simulink model "initial_setup"  (R2012b)
settings: Solver=FixedStepDiscrete  StartTime=0.0  StopTime=inf  FixedStep=sample_time  RelTol=1e-3
InitFcn:
  | init_initial_setup;
values from neighbouring files (symbols this model uses):
  fcut_unwrap = 50    [init_initial_setup.m]
  fcut_velocity = 100    [init_initial_setup.m]
  sample_time = 1/update_freq    (= 0.001)    [init_initial_setup.m]
undefined symbols (not defined in the file or in its folder): A_angle_h, A_angle_k, A_angle_lat, angle_midpoint_h, angle_midpoint_k, angle_midpoint_lat, BOOM_MAX_ENCODER_TICKS, BOOM_PITCH_CAL_VALUE_RAD, BOOM_PITCH_CAL_VALUE_TICKS, BOOM_PITCH_ENCODER_RAD_PER_TICK, BOOM_ROLL_CAL_VALUE_RAD, BOOM_ROLL_CAL_VALUE_TICKS, BOOM_ROLL_ENCODER_RAD_PER_TICK, BOOM_YAW_ENCODER_RAD_PER_TICK, control_start_time, HIP_ABS_ENCODER_RAD_PER_TICK, HIP_INC_ENCODER_RAD_PER_TICK, HIP_INC_MAX_ENCODER_TICKS, k_leg_spring, kd_h_sine_walk, kd_k_sine_walk, kd_lat, kd_sea_position, kd_sea_torque, kd_velocity, kp_h_sine_walk, kp_k_sine_walk, kp_lat, kp_sea_position, kp_sea_torque, kp_velocity, LEFT_HIP_CALIB_POS, LEFT_HIP_CALIB_VAL, LEFT_MOTOR_HIP_DIRECTION, LEG1_LEG_A_CALIB_VAL, LEG1_LEG_A_RAD_PER_CNT, LEG1_LEG_B_CALIB_VAL, LEG1_LEG_B_RAD_PER_CNT, LEG1_MOTOR_A_DIRECTION, LEG1_MOTOR_B_DIRECTION, LEG1_TRAN_A_CALIB_VAL, LEG1_TRAN_A_RAD_PER_CNT, LEG1_TRAN_B_CALIB_VAL, LEG1_TRAN_B_RAD_PER_CNT, LEG2_LEG_A_CALIB_VAL, LEG2_LEG_A_RAD_PER_CNT, LEG2_LEG_B_CALIB_VAL, LEG2_LEG_B_RAD_PER_CNT, LEG2_MOTOR_A_DIRECTION, LEG2_MOTOR_B_DIRECTION, LEG2_TRAN_A_CALIB_VAL, LEG2_TRAN_A_RAD_PER_CNT, LEG2_TRAN_B_CALIB_VAL, LEG2_TRAN_B_RAD_PER_CNT, LEG_A_CALIB_LOC, LEG_B_CALIB_LOC, LEG_MTR_GEAR_RATIO, LEG_MTR_MAX_TORQUE, LEG_MTR_MAX_VELOCITY, MTR_HIP_MAX_CURRENT ... (+10)
libraries: xpcethercatlib x160, simulink x34, dspswit3 x1
(part 3 of 4)

== system initial_setup/Simple Sinusoidal Motion/SEA Controllers (Left Leg) ==
  phi_load_back : Inport
  phi_gear_back : Inport  Port=2
  phi_load_front : Inport  Port=3
  phi_gear_front : Inport  Port=4
  tau_des_back : Inport  Port=5
  tau_des_front : Inport  Port=6
  SEA Controller (Position) back : Subsystem
  SEA Controller (Position) front : Subsystem
  SEA Controller (Velocity) back : Subsystem  Commented=on
  SEA Controller (Velocity) front : Subsystem  Commented=on
  tau_cmd_back : Outport
  tau_cmd_front : Outport  Port=2
  wires:
  phi_load_front/1 -> SEA Controller (Position) front/1(phi_load [rad])
  tau_des_front/1 -> SEA Controller (Position) front/3(tau_des [Nm])
  SEA Controller (Position) back/1(tau_cmd [Nm]) -> tau_cmd_back/1
  phi_gear_back/1 -> SEA Controller (Position) back/2(phi_gear [rad])
  phi_gear_front/1 -> SEA Controller (Position) front/2(phi_gear [rad])
  phi_load_back/1 -> SEA Controller (Position) back/1(phi_load [rad])
  tau_des_back/1 -> SEA Controller (Position) back/3(tau_des [Nm])
  SEA Controller (Position) front/1(tau_cmd [Nm]) -> tau_cmd_front/1

== system initial_setup/Simple Sinusoidal Motion/SEA Controllers (Right Leg) ==
  phi_load_back : Inport
  phi_gear_back : Inport  Port=2
  phi_load_front : Inport  Port=3
  phi_gear_front : Inport  Port=4
  tau_des_back : Inport  Port=5
  tau_des_front : Inport  Port=6
  SEA Controller (Position) back : Subsystem
  SEA Controller (Position) front : Subsystem
  SEA Controller (Velocity) back : Subsystem  Commented=on
  SEA Controller (Velocity) front : Subsystem  Commented=on
  tau_cmd_back : Outport
  tau_cmd_front : Outport  Port=2
  wires:
  SEA Controller (Position) front/1(tau_cmd [Nm]) -> tau_cmd_front/1
  tau_des_back/1 -> SEA Controller (Position) back/3(tau_des [Nm])
  phi_load_back/1 -> SEA Controller (Position) back/1(phi_load [rad])
  phi_gear_front/1 -> SEA Controller (Position) front/2(phi_gear [rad])
  phi_gear_back/1 -> SEA Controller (Position) back/2(phi_gear [rad])
  SEA Controller (Position) back/1(tau_cmd [Nm]) -> tau_cmd_back/1
  tau_des_front/1 -> SEA Controller (Position) front/3(tau_des [Nm])
  phi_load_front/1 -> SEA Controller (Position) front/1(phi_load [rad])

== system initial_setup/DAQ/calibrate_and_convert_to_rad/calibrate_abs_encoder ==
  encoder_ticks : Inport
  cal_pt_ticks : Inport  Port=2
  cal_pt_rad : Inport  Port=3
  ticks_to_rad_const : Inport  Port=4
  Product : Product  RndMeth=Zero
  Sum : Sum  Inputs=|+-
  Sum1 : Sum  Inputs=|++
  angle [rad] : Outport
  wires:
  cal_pt_rad/1 -> Sum1/2  "calibration_point_radians"
  Sum1/1 -> angle [rad]/1  "calibrated_angle"
  cal_pt_ticks/1 -> Sum/2  "calibration_point_ticks"
  ticks_to_rad_const/1 -> Product/2  "ticks_to_rad_const"
  Product/1 -> Sum1/1  "rad_diff"
  encoder_ticks/1 -> Sum/1  "encoder_ticks"
  Sum/1 -> Product/1  "tick_diff"

== system initial_setup/DAQ/calibrate_and_convert_to_rad/calibration_pt_radians ==
  Constant{1,3,5,7} (4 alike) : Constant  Value=LEG_A_CALIB_LOC
  Constant10 : Constant  Value=LEFT_HIP_CALIB_POS
  Constant11 : Constant  Value=BOOM_ROLL_CAL_VALUE_RAD
  Constant12 : Constant  Value=BOOM_PITCH_CAL_VALUE_RAD
  Constant{2,4,6,8} (4 alike) : Constant  Value=LEG_B_CALIB_LOC
  Constant9 : Constant  Value=RIGHT_HIP_CALIB_POS
  Mux3 : Mux  Inputs=12
  calibration_pt [rad] : Outport
  wires:
  Constant7/1 -> Mux3/5
  Constant10/1 -> Mux3/9
  Constant1/1 -> Mux3/2
  Constant5/1 -> Mux3/6
  Constant2/1 -> Mux3/3
  Constant9/1 -> Mux3/10
  Constant12/1 -> Mux3/12
  Constant6/1 -> Mux3/7
  Constant11/1 -> Mux3/11
  Mux3/1 -> calibration_pt [rad]/1
  Constant3/1 -> Mux3/1
  Constant8/1 -> Mux3/8
  Constant4/1 -> Mux3/4

== system initial_setup/DAQ/calibrate_and_convert_to_rad/calibration_pt_ticks ==
  Constant1 : Constant  Value=LEG2_TRAN_A_CALIB_VAL
  Constant10 : Constant  Value=LEFT_HIP_CALIB_VAL
  Constant11 : Constant  Value=BOOM_ROLL_CAL_VALUE_TICKS
  Constant12 : Constant  Value=BOOM_PITCH_CAL_VALUE_TICKS
  Constant2 : Constant  Value=LEG2_LEG_B_CALIB_VAL
  Constant3 : Constant  Value=LEG2_LEG_A_CALIB_VAL
  Constant4 : Constant  Value=LEG2_TRAN_B_CALIB_VAL
  Constant5 : Constant  Value=LEG1_TRAN_A_CALIB_VAL
  Constant6 : Constant  Value=LEG1_LEG_B_CALIB_VAL
  Constant7 : Constant  Value=LEG1_LEG_A_CALIB_VAL
  Constant8 : Constant  Value=LEG1_TRAN_B_CALIB_VAL
  Constant9 : Constant  Value=RIGHT_HIP_CALIB_VAL
  Mux3 : Mux  Inputs=12
  calibration_pt [ticks] : Outport
  wires:
  Constant8/1 -> Mux3/4
  Constant4/1 -> Mux3/8
  Constant7/1 -> Mux3/1
  Mux3/1 -> calibration_pt [ticks]/1
  Constant11/1 -> Mux3/11
  Constant2/1 -> Mux3/7
  Constant12/1 -> Mux3/12
  Constant9/1 -> Mux3/10
  Constant6/1 -> Mux3/3
  Constant1/1 -> Mux3/6
  Constant5/1 -> Mux3/2
  Constant10/1 -> Mux3/9
  Constant3/1 -> Mux3/5

== system initial_setup/DAQ/calibrate_and_convert_to_rad/ticks_to_radians_constants ==
  Constant1 : Constant  Value=LEG2_TRAN_A_RAD_PER_CNT
  Constant10 : Constant  Value=-HIP_ABS_ENCODER_RAD_PER_TICK
  Constant11 : Constant  Value=BOOM_ROLL_ENCODER_RAD_PER_TICK
  Constant12 : Constant  Value=BOOM_PITCH_ENCODER_RAD_PER_TICK
  Constant2 : Constant  Value=LEG2_LEG_B_RAD_PER_CNT
  Constant3 : Constant  Value=LEG2_LEG_A_RAD_PER_CNT
  Constant4 : Constant  Value=LEG2_TRAN_B_RAD_PER_CNT
  Constant5 : Constant  Value=LEG1_TRAN_A_RAD_PER_CNT
  Constant6 : Constant  Value=LEG1_LEG_B_RAD_PER_CNT
  Constant7 : Constant  Value=LEG1_LEG_A_RAD_PER_CNT
  Constant8 : Constant  Value=LEG1_TRAN_B_RAD_PER_CNT
  Constant9 : Constant  Value=HIP_ABS_ENCODER_RAD_PER_TICK
  Mux3 : Mux  Inputs=12
  ticks_to_rad_constants : Outport
  wires:
  Constant8/1 -> Mux3/4
  Constant4/1 -> Mux3/8
  Constant7/1 -> Mux3/1
  Mux3/1 -> ticks_to_rad_constants/1
  Constant11/1 -> Mux3/11
  Constant2/1 -> Mux3/7
  Constant12/1 -> Mux3/12
  Constant10/1 -> Mux3/10
  Constant6/1 -> Mux3/3
  Constant1/1 -> Mux3/6
  Constant5/1 -> Mux3/2
  Constant9/1 -> Mux3/9
  Constant3/1 -> Mux3/5

== system initial_setup/DAQ/hold_initial_lateral_angles/Initial Lateral Hip Angles [rad] ==
  In : Inport
  Enable : EnablePort  StatesWhenEnabling=reset
  Out : Outport
  wires:
  In/1 -> Out/1

== system initial_setup/DAQ/unwrap_encoders/unwrap_boom_yaw_encoder ==
  note: predicted angle:
      | phi' = phi_(n-1) + dphi
      | = phi_(n-1) + phi_(n-1)-phi_(n-2)
  note: Transform Wrapped Angle into Continuous Angle
  note: Recommended if-then structure for assigning
      | constants. The criterion '~=0' is realized as cpu register
      | shift when compiling.  The resulting code is fast.
  wrapped [ticks] : Inport
  1/BOOM_MAX_ENCODER_TICKS : Gain  Gain=1/BOOM_MAX_ENCODER_TICKS
  Abs : Abs
  BOOM_MAX_ENCODER_TICKS : Gain  Gain=BOOM_MAX_ENCODER_TICKS
  Compare To Zero : simulink/Logic and Bit Operations/Compare To Zero  relop=>  OutDataTypeStr=uint8
  Discrete Single Pole Lowpass Filter : DiscreteTransferFcn  Numerator=[(1-exp(-2*pi*fcut_unwrap*sample_time)) 0]  Denominator=[1 -exp(-2*pi*fcut_unwrap*sample_time)]  SampleTime=sample_time
  Gain2 : Gain  Gain=2
  Product : Product  RndMeth=Zero
  Rounding Function : Rounding
  Sum : Sum  Inputs=|+-
  Sum1 : Sum  Inputs=|++
  Sum2 : Sum  Inputs=|++
  Sum3 : Sum  Inputs=-+|
  Switch : Switch  Criteria=u2 ~= 0
      settings: AttributesFormatString=%<Criteria>
  Unit Delay phi_(n-1) : UnitDelay  SampleTime=-1
      settings: AttributesFormatString=initial condition = %<X0>
  Unit Delay phi_(n-2) : UnitDelay  SampleTime=-1
      settings: AttributesFormatString=initial condition = %<X0>
  const : Constant  Value=0.5
  no : Constant  Value=-1
  yes : Constant
  continuous [ticks] : Outport
  wires:
  Sum3/1 -> Compare To Zero/1, Abs/1  "phi'-phi"
  Sum/1 -> Sum3/2
  Gain2/1 -> Sum/1
  Unit Delay phi_(n-1)/1 -> Gain2/1, Unit Delay phi_(n-2)/1
  BOOM_MAX_ENCODER_TICKS/1 -> Product/1
  Sum1/1 -> Discrete Single Pole Lowpass Filter/1, continuous [ticks]/1
  Sum2/1 -> Rounding Function/1
  const/1 -> Sum2/2
  1/BOOM_MAX_ENCODER_TICKS/1 -> Sum2/1
  Abs/1 -> 1/BOOM_MAX_ENCODER_TICKS/1
  Product/1 -> Sum1/2
  wrapped [ticks]/1 -> Sum3/1, Sum1/1
  Rounding Function/1 -> BOOM_MAX_ENCODER_TICKS/1
  Switch/1 -> Product/2
  no/1 -> Switch/3
  yes/1 -> Switch/1
  Unit Delay phi_(n-2)/1 -> Sum/2
  Compare To Zero/1 -> Switch/2
  Discrete Single Pole Lowpass Filter/1 -> Unit Delay phi_(n-1)/1

== system initial_setup/DAQ/unwrap_encoders/unwrap_lateral_incremental_encoders Left ==
  note: predicted angle:
      | phi' = phi_(n-1) + dphi
      | = phi_(n-1) + phi_(n-1)-phi_(n-2)
  note: Transform Wrapped Angle into Continuous Angle
  note: Recommended if-then structure for assigning
      | constants. The criterion '~=0' is realized as cpu register
      | shift when compiling.  The resulting code is fast.
  wrapped [ticks] : Inport
  1/HIP_INC_MAX_ENCODER_TICKS : Gain  Gain=1/HIP_INC_MAX_ENCODER_TICKS
  Abs : Abs
  Compare To Zero : simulink/Logic and Bit Operations/Compare To Zero  relop=>  OutDataTypeStr=uint8
  Discrete Single Pole Lowpass Filter : DiscreteTransferFcn  Numerator=[(1-exp(-2*pi*fcut_unwrap*sample_time)) 0]  Denominator=[1 -exp(-2*pi*fcut_unwrap*sample_time)]  SampleTime=sample_time
  Gain2 : Gain  Gain=2
  HIP_INC_MAX_ENCODER_TICKS : Gain  Gain=HIP_INC_MAX_ENCODER_TICKS
  Product : Product  RndMeth=Zero
  Rounding Function : Rounding
  Sum : Sum  Inputs=|+-
  Sum1 : Sum  Inputs=|++
  Sum2 : Sum  Inputs=|++
  Sum3 : Sum  Inputs=-+|
  Switch : Switch  Criteria=u2 ~= 0
      settings: AttributesFormatString=%<Criteria>
  Unit Delay phi_(n-1) : UnitDelay  SampleTime=-1
      settings: AttributesFormatString=initial condition = %<X0>
  Unit Delay phi_(n-2) : UnitDelay  SampleTime=-1
      settings: AttributesFormatString=initial condition = %<X0>
  const : Constant  Value=0.5
  no : Constant  Value=-1
  yes : Constant
  continuous [ticks] : Outport
  wires:
  Sum3/1 -> Compare To Zero/1, Abs/1  "phi'-phi"
  Sum/1 -> Sum3/2
  Gain2/1 -> Sum/1
  Unit Delay phi_(n-1)/1 -> Gain2/1, Unit Delay phi_(n-2)/1
  HIP_INC_MAX_ENCODER_TICKS/1 -> Product/1
  Sum1/1 -> continuous [ticks]/1, Discrete Single Pole Lowpass Filter/1
  Sum2/1 -> Rounding Function/1
  const/1 -> Sum2/2
  1/HIP_INC_MAX_ENCODER_TICKS/1 -> Sum2/1
  Abs/1 -> 1/HIP_INC_MAX_ENCODER_TICKS/1
  Product/1 -> Sum1/2
  wrapped [ticks]/1 -> Sum3/1, Sum1/1
  Rounding Function/1 -> HIP_INC_MAX_ENCODER_TICKS/1
  Switch/1 -> Product/2
  no/1 -> Switch/3
  yes/1 -> Switch/1
  Unit Delay phi_(n-2)/1 -> Sum/2
  Compare To Zero/1 -> Switch/2
  Discrete Single Pole Lowpass Filter/1 -> Unit Delay phi_(n-1)/1

== system initial_setup/DAQ/unwrap_encoders/unwrap_lateral_incremental_encoders Right ==
  note: Recommended if-then structure for assigning
      | constants. The criterion '~=0' is realized as cpu register
      | shift when compiling.  The resulting code is fast.
  note: Transform Wrapped Angle into Continuous Angle
  note: predicted angle:
      | phi' = phi_(n-1) + dphi
      | = phi_(n-1) + phi_(n-1)-phi_(n-2)
  wrapped [ticks] : Inport
  1/HIP_INC_MAX_ENCODER_TICKS : Gain  Gain=1/HIP_INC_MAX_ENCODER_TICKS
  Abs : Abs
  Compare To Zero : simulink/Logic and Bit Operations/Compare To Zero  relop=>  OutDataTypeStr=uint8
  Discrete Single Pole Lowpass Filter : DiscreteTransferFcn  Numerator=[(1-exp(-2*pi*fcut_unwrap*sample_time)) 0]  Denominator=[1 -exp(-2*pi*fcut_unwrap*sample_time)]  SampleTime=sample_time
  Gain2 : Gain  Gain=2
  HIP_INC_MAX_ENCODER_TICKS : Gain  Gain=HIP_INC_MAX_ENCODER_TICKS
  Product : Product  RndMeth=Zero
  Rounding Function : Rounding
  Sum : Sum  Inputs=|+-
  Sum1 : Sum  Inputs=|++
  Sum2 : Sum  Inputs=|++
  Sum3 : Sum  Inputs=-+|
  Switch : Switch  Criteria=u2 ~= 0
      settings: AttributesFormatString=%<Criteria>
  Unit Delay phi_(n-1) : UnitDelay  SampleTime=-1
      settings: AttributesFormatString=initial condition = %<X0>
  Unit Delay phi_(n-2) : UnitDelay  SampleTime=-1
      settings: AttributesFormatString=initial condition = %<X0>
  const : Constant  Value=0.5
  no : Constant  Value=-1
  yes : Constant
  continuous [ticks] : Outport
  wires:
  Discrete Single Pole Lowpass Filter/1 -> Unit Delay phi_(n-1)/1
  Compare To Zero/1 -> Switch/2
  Unit Delay phi_(n-2)/1 -> Sum/2
  yes/1 -> Switch/1
  no/1 -> Switch/3
  Switch/1 -> Product/2
  Rounding Function/1 -> HIP_INC_MAX_ENCODER_TICKS/1
  wrapped [ticks]/1 -> Sum1/1, Sum3/1
  Product/1 -> Sum1/2
  Abs/1 -> 1/HIP_INC_MAX_ENCODER_TICKS/1
  1/HIP_INC_MAX_ENCODER_TICKS/1 -> Sum2/1
  const/1 -> Sum2/2
  Sum2/1 -> Rounding Function/1
  Sum1/1 -> Discrete Single Pole Lowpass Filter/1, continuous [ticks]/1
  HIP_INC_MAX_ENCODER_TICKS/1 -> Product/1
  Unit Delay phi_(n-1)/1 -> Unit Delay phi_(n-2)/1, Gain2/1
  Gain2/1 -> Sum/1
  Sum/1 -> Sum3/2
  Sum3/1 -> Abs/1, Compare To Zero/1  "phi'-phi"

== system initial_setup/Simple Sinusoidal Motion/Left Lateral Sine Wave/Diminish ==
  desQ : Inport
  Clock : Clock
  Divide : Product  Inputs=*/
  Position Saturation : Saturate  UpperLimit=0  LowerLimit=-5*pi/180
  Ramp : simulink/Sources/Ramp  slope=pi/10  start=t_lat  X0=1
  Ramp1 : simulink/Sources/Ramp  slope=-0.5*pi/180  start=t_lat  X0=0
  Sum : Sum  Inputs=++|
  Switch : Switch  Threshold=t_lat
  desQ' : Outport
  wires:
  Clock/1 -> Switch/2
  Ramp/1 -> Divide/2
  Switch/1 -> desQ'/1
  desQ/1 -> Switch/3, Divide/1
  Ramp1/1 -> Position Saturation/1
  Divide/1 -> Sum/2
  Position Saturation/1 -> Sum/1
  Sum/1 -> Switch/1

== system initial_setup/Simple Sinusoidal Motion/Left Lateral Sine Wave/Hip Roll PD ==
  Desired Position / Velocity : Inport
  Position / Velocity : Inport  Port=2
  Demux : Demux  Outputs=2
  Demux1 : Demux  Outputs=2
  Gain4 : Gain  Gain=kp_lat
  Gain5 : Gain  Gain=kd_lat
  Sum4 : Sum  Inputs=|+-
  Sum5 : Sum  Inputs=|+-
  Sum6 : Sum  Inputs=|++
  tauLat : Outport
  wires:
  Sum6/1 -> tauLat/1
  Demux/1 -> Sum4/2  "position"
  Position / Velocity/1 -> Demux/1
  Sum4/1 -> Gain4/1
  Sum5/1 -> Gain5/1
  Gain4/1 -> Sum6/1
  Demux/2 -> Sum5/2  "velocity"
  Gain5/1 -> Sum6/2
  Demux1/2 -> Sum5/1
  Desired Position / Velocity/1 -> Demux1/1
  Demux1/1 -> Sum4/1

== system initial_setup/Simple Sinusoidal Motion/Left Leg Sagittal Sine Wave/Hip PD Torque Control ==
  Desired Angle : Inport
  Desired Velocity : Inport  Port=2
  Hip Position / Velocity : Inport  Port=3
  Demux : Demux  Outputs=2
  Gain4 : Gain  Gain=kp_h_sine_walk
  Gain5 : Gain  Gain=kd_h_sine_walk
  Sum4 : Sum  Inputs=|+-
  Sum5 : Sum  Inputs=|+-
  Sum6 : Sum  Inputs=|++
  Tau Hip : Outport
  wires:
  Gain5/1 -> Sum6/2
  Demux/2 -> Sum5/2  "theta_h_dot_measured"
  Gain4/1 -> Sum6/1
  Sum5/1 -> Gain5/1
  Sum4/1 -> Gain4/1
  Desired Velocity/1 -> Sum5/1
  Hip Position / Velocity/1 -> Demux/1
  Demux/1 -> Sum4/2  "theta_h_measured"
  Desired Angle/1 -> Sum4/1
  Sum6/1 -> Tau Hip/1

== system initial_setup/Simple Sinusoidal Motion/Left Leg Sagittal Sine Wave/Knee PD Torque Control ==
  Desired Angle : Inport
  Desired Velocity : Inport  Port=2
  Knee Position / Velocity : Inport  Port=3
  Demux1 : Demux  Outputs=2
  Gain6 : Gain  Gain=kp_k_sine_walk
  Gain7 : Gain  Gain=kd_k_sine_walk
  Sum7 : Sum  Inputs=|+-
  Sum8 : Sum  Inputs=|+-
  Sum9 : Sum  Inputs=|++
  Tau Knee : Outport
  wires:
  Gain6/1 -> Sum9/1
  Gain7/1 -> Sum9/2
  Knee Position / Velocity/1 -> Demux1/1
  Demux1/2 -> Sum8/2  "theta_k_dot_measured"
  Desired Angle/1 -> Sum7/1
  Sum8/1 -> Gain7/1
  Desired Velocity/1 -> Sum8/1
  Sum9/1 -> Tau Knee/1
  Demux1/1 -> Sum7/2  "theta_k_measured"
  Sum7/1 -> Gain6/1

== system initial_setup/Simple Sinusoidal Motion/Right Lateral Sine Wave/Diminish ==
  desQ : Inport
  Clock : Clock
  Divide : Product  Inputs=*/
  Position Saturation : Saturate  UpperLimit=0  LowerLimit=-5*pi/180
  Ramp : simulink/Sources/Ramp  slope=-0.5*pi/180  start=t_lat  X0=0
  Ramp1 : simulink/Sources/Ramp  slope=pi/10  start=t_lat  X0=1
  Sum : Sum  Inputs=++|
  Switch : Switch  Threshold=t_lat
  desQ' : Outport
  wires:
  Clock/1 -> Switch/2
  Ramp1/1 -> Divide/2
  Switch/1 -> desQ'/1
  desQ/1 -> Switch/3, Divide/1
  Ramp/1 -> Position Saturation/1
  Divide/1 -> Sum/2
  Sum/1 -> Switch/1
  Position Saturation/1 -> Sum/1

== system initial_setup/Simple Sinusoidal Motion/Right Lateral Sine Wave/Hip Roll PD ==
  Desired Position / Velocity : Inport
  Position / Velocity : Inport  Port=2
  Demux : Demux  Outputs=2
  Demux1 : Demux  Outputs=2
  Gain4 : Gain  Gain=kp_lat
  Gain5 : Gain  Gain=kd_lat
  Sum4 : Sum  Inputs=|+-
  Sum5 : Sum  Inputs=|+-
  Sum6 : Sum  Inputs=|++
  tauLat : Outport
  wires:
  Gain5/1 -> Sum6/2
  Demux/2 -> Sum5/2  "velocity"
  Gain4/1 -> Sum6/1
  Sum5/1 -> Gain5/1
  Sum4/1 -> Gain4/1
  Demux1/2 -> Sum5/1
  Position / Velocity/1 -> Demux/1
  Demux/1 -> Sum4/2  "position"
  Desired Position / Velocity/1 -> Demux1/1
  Sum6/1 -> tauLat/1
  Demux1/1 -> Sum4/1

== system initial_setup/Simple Sinusoidal Motion/Right Leg Sagittal Sine Wave/Hip PD Torque Control ==
  Desired Angle : Inport
  Desired Velocity : Inport  Port=2
  Hip Position / Velocity : Inport  Port=3
  Demux : Demux  Outputs=2
  Gain4 : Gain  Gain=kp_h_sine_walk
  Gain5 : Gain  Gain=kd_h_sine_walk
  Sum4 : Sum  Inputs=|+-
  Sum5 : Sum  Inputs=|+-
  Sum6 : Sum  Inputs=|++
  Tau Hip : Outport
  wires:
  Sum6/1 -> Tau Hip/1
  Desired Angle/1 -> Sum4/1
  Demux/1 -> Sum4/2  "theta_h_measured"
  Hip Position / Velocity/1 -> Demux/1
  Desired Velocity/1 -> Sum5/1
  Sum4/1 -> Gain4/1
  Sum5/1 -> Gain5/1
  Gain4/1 -> Sum6/1
  Demux/2 -> Sum5/2  "theta_h_dot_measured"
  Gain5/1 -> Sum6/2

== system initial_setup/Simple Sinusoidal Motion/Right Leg Sagittal Sine Wave/Knee PD Torque Control ==
  Desired Angle : Inport
  Desired Velocity : Inport  Port=2
  Knee Position / Velocity : Inport  Port=3
  Demux1 : Demux  Outputs=2
  Gain6 : Gain  Gain=kp_k_sine_walk
  Gain7 : Gain  Gain=kd_k_sine_walk
  Sum7 : Sum  Inputs=|+-
  Sum8 : Sum  Inputs=|+-
  Sum9 : Sum  Inputs=|++
  Tau Knee : Outport
  wires:
  Sum7/1 -> Gain6/1
  Demux1/1 -> Sum7/2  "theta_k_measured"
  Sum9/1 -> Tau Knee/1
  Desired Velocity/1 -> Sum8/1
  Sum8/1 -> Gain7/1
  Desired Angle/1 -> Sum7/1
  Demux1/2 -> Sum8/2  "theta_k_dot_measured"
  Knee Position / Velocity/1 -> Demux1/1
  Gain7/1 -> Sum9/2
  Gain6/1 -> Sum9/1

== system initial_setup/Simple Sinusoidal Motion/SEA Controllers (Left Leg)/SEA Controller (Position) back ==
  phi_load [rad] : Inport
  phi_gear [rad] : Inport  Port=2
  tau_des [Nm] : Inport  Port=3
  Gain2 : Gain  Gain=1/k_leg_spring
  Position PD : Subsystem
  Spring Stiffness : Gain  Gain=k_leg_spring
  Sum1 : Sum  Inputs=+-
  Sum2 : Sum  Inputs=|+-
  Sum3 : Sum  Inputs=+|+
  Sum4 : Sum  Inputs=|+-
  Sum5 : Sum  Inputs=++|
  "Torque Limiter (outside) " : Saturate  UpperLimit=LEG_MTR_MAX_TORQUE  LowerLimit=-LEG_MTR_MAX_TORQUE
  Torque PD : Subsystem
  tau_cmd [Nm] : Outport
  wires:
  phi_gear [rad]/1 -> Sum1/1, Sum4/2
  Sum4/1 -> Position PD/1(position_Err)
  Position PD/1(out) -> tau_cmd [Nm]/1
  "Torque Limiter (outside) "/1 -> Sum2/1, Gain2/1
  Gain2/1 -> Sum3/1
  Spring Stiffness/1 -> Sum2/2  "tau_L"
  tau_des [Nm]/1 -> "Torque Limiter (outside) "/1
  Sum2/1 -> Torque PD/1(tau_Err)  "tau_Err"
  Sum1/1 -> Spring Stiffness/1
  phi_load [rad]/1 -> Sum3/2, Sum1/2
  Sum3/1 -> Sum5/1
  Sum5/1 -> Sum4/1
  Torque PD/1(out) -> Sum5/2

== system initial_setup/Simple Sinusoidal Motion/SEA Controllers (Left Leg)/SEA Controller (Position) front ==
  phi_load [rad] : Inport
  phi_gear [rad] : Inport  Port=2
  tau_des [Nm] : Inport  Port=3
  Gain2 : Gain  Gain=1/k_leg_spring
  Position PD : Subsystem
  Spring Stiffness : Gain  Gain=k_leg_spring
  Sum1 : Sum  Inputs=+-
  Sum2 : Sum  Inputs=|+-
  Sum3 : Sum  Inputs=+|+
  Sum4 : Sum  Inputs=|+-
  Sum5 : Sum  Inputs=++|
  "Torque Limiter (outside) " : Saturate  UpperLimit=LEG_MTR_MAX_TORQUE  LowerLimit=-LEG_MTR_MAX_TORQUE
  Torque PD : Subsystem
  tau_cmd [Nm] : Outport
  wires:
  Torque PD/1(out) -> Sum5/2
  Sum5/1 -> Sum4/1
  Sum3/1 -> Sum5/1
  phi_load [rad]/1 -> Sum1/2, Sum3/2
  Sum1/1 -> Spring Stiffness/1
  Sum2/1 -> Torque PD/1(tau_Err)  "tau_Err"
  tau_des [Nm]/1 -> "Torque Limiter (outside) "/1
  Spring Stiffness/1 -> Sum2/2  "tau_L"
  Gain2/1 -> Sum3/1
  "Torque Limiter (outside) "/1 -> Gain2/1, Sum2/1
  Position PD/1(out) -> tau_cmd [Nm]/1
  Sum4/1 -> Position PD/1(position_Err)
  phi_gear [rad]/1 -> Sum4/2, Sum1/1

== system initial_setup/Simple Sinusoidal Motion/SEA Controllers (Left Leg)/SEA Controller (Velocity) back ==
  note: Feedback Error Compensation
  note: SEA
      | Electromechanical
      | Process
      | Dynamics
  note: Inverse Dynamics Compensation
  note: Anticipatory Feedforward Compensation
  phi_load [rad] : Inport
  phi_gear [rad] : Inport  Port=2
  tau_des [Nm] : Inport  Port=3
  1st Lead Compensator : Subsystem
  Gain2 : Gain  Gain=1/k_leg_spring
  Gear Ratio2 : Gain  Gain=LEG_MTR_GEAR_RATIO
  Lead Compensator : Subsystem
  PD : Subsystem
  PID : Subsystem
  Spring Stiffness : Gain  Gain=k_leg_spring
  Sum1 : Sum  Inputs=+-
  Sum2 : Sum  Inputs=|+-
  Sum3 : Sum  Inputs=+|+
  Sum4 : Sum  Inputs=|+-
  Sum5 : Sum  Inputs=++|
  "Torque Limiter (outside) " : Saturate  UpperLimit=LEG_MTR_MAX_TORQUE  LowerLimit=-LEG_MTR_MAX_TORQUE
  Velocity Limiter : Saturate  UpperLimit=LEG_MTR_MAX_VELOCITY  LowerLimit=-LEG_MTR_MAX_VELOCITY
  filtered_derivative : Subsystem
  tau_cmd [Nm] : Outport
  wires:
  PD/1(tau_mtr [Nm]) -> tau_cmd [Nm]/1
  Sum3/1 -> Sum5/1
  Gear Ratio2/1 -> Sum4/2
  filtered_derivative/1(dx/dt) -> Gear Ratio2/1
  Sum4/1 -> PD/1(velocity_err [rad/s])
  Velocity Limiter/1 -> Sum4/1
  Lead Compensator/1(dx/dt) -> Sum3/2
  "Torque Limiter (outside) "/1 -> Gain2/1, Sum2/1
  Sum5/1 -> Velocity Limiter/1  "dphi_gearhead_des  [m/s]"
  phi_gear [rad]/1 -> Sum1/1, filtered_derivative/1(x)
  1st Lead Compensator/1(dx/dt) -> Sum3/1
  PID/1("dphi_gearhead_des [rad/s] ") -> Sum5/2
  Spring Stiffness/1 -> Sum2/2  "tau_L"
  tau_des [Nm]/1 -> "Torque Limiter (outside) "/1
  Sum2/1 -> PID/1(tau_Err)  "tau_Err"
  Sum1/1 -> Spring Stiffness/1
  phi_load [rad]/1 -> Sum1/2, Lead Compensator/1(x)
  Gain2/1 -> 1st Lead Compensator/1(x)

== system initial_setup/Simple Sinusoidal Motion/SEA Controllers (Left Leg)/SEA Controller (Velocity) front ==
  note: Anticipatory Feedforward Compensation
  note: Inverse Dynamics Compensation
  note: SEA
      | Electromechanical
      | Process
      | Dynamics
  note: Feedback Error Compensation
  phi_load [rad] : Inport
  phi_gear [rad] : Inport  Port=2
  tau_des [Nm] : Inport  Port=3
  1st Lead Compensator : Subsystem
  Gain2 : Gain  Gain=1/k_leg_spring
  Gear Ratio2 : Gain  Gain=LEG_MTR_GEAR_RATIO
  Lead Compensator : Subsystem
  PD : Subsystem
  PID : Subsystem
  Spring Stiffness : Gain  Gain=k_leg_spring
  Sum1 : Sum  Inputs=+-
  Sum2 : Sum  Inputs=|+-
  Sum3 : Sum  Inputs=+|+
  Sum4 : Sum  Inputs=|+-
  Sum5 : Sum  Inputs=++|
  "Torque Limiter (outside) " : Saturate  UpperLimit=LEG_MTR_MAX_TORQUE  LowerLimit=-LEG_MTR_MAX_TORQUE
  Velocity Limiter : Saturate  UpperLimit=LEG_MTR_MAX_VELOCITY  LowerLimit=-LEG_MTR_MAX_VELOCITY
  filtered_derivative : Subsystem
  tau_cmd [Nm] : Outport
  wires:
  Gain2/1 -> 1st Lead Compensator/1(x)
  phi_load [rad]/1 -> Lead Compensator/1(x), Sum1/2
  Sum1/1 -> Spring Stiffness/1
  Sum2/1 -> PID/1(tau_Err)  "tau_Err"
  tau_des [Nm]/1 -> "Torque Limiter (outside) "/1
  Spring Stiffness/1 -> Sum2/2  "tau_L"
  PID/1("dphi_gearhead_des [rad/s] ") -> Sum5/2
  1st Lead Compensator/1(dx/dt) -> Sum3/1
  phi_gear [rad]/1 -> filtered_derivative/1(x), Sum1/1
  Sum5/1 -> Velocity Limiter/1  "dphi_gearhead_des  [m/s]"
  "Torque Limiter (outside) "/1 -> Sum2/1, Gain2/1
  Lead Compensator/1(dx/dt) -> Sum3/2
  Velocity Limiter/1 -> Sum4/1
  Sum4/1 -> PD/1(velocity_err [rad/s])
  filtered_derivative/1(dx/dt) -> Gear Ratio2/1
  Gear Ratio2/1 -> Sum4/2
  Sum3/1 -> Sum5/1
  PD/1(tau_mtr [Nm]) -> tau_cmd [Nm]/1

== system initial_setup/Simple Sinusoidal Motion/SEA Controllers (Right Leg)/SEA Controller (Position) back ==
  phi_load [rad] : Inport
  phi_gear [rad] : Inport  Port=2
  tau_des [Nm] : Inport  Port=3
  Gain2 : Gain  Gain=1/k_leg_spring
  Position PD : Subsystem
  Spring Stiffness : Gain  Gain=k_leg_spring
  Sum1 : Sum  Inputs=+-
  Sum2 : Sum  Inputs=|+-
  Sum3 : Sum  Inputs=+|+
  Sum4 : Sum  Inputs=|+-
  Sum5 : Sum  Inputs=++|
  "Torque Limiter (outside) " : Saturate  UpperLimit=LEG_MTR_MAX_TORQUE  LowerLimit=-LEG_MTR_MAX_TORQUE
  Torque PD : Subsystem
  tau_cmd [Nm] : Outport
  wires:
  Torque PD/1(out) -> Sum5/2
  Sum5/1 -> Sum4/1
  Sum3/1 -> Sum5/1
  phi_load [rad]/1 -> Sum1/2, Sum3/2
  Sum1/1 -> Spring Stiffness/1
  Sum2/1 -> Torque PD/1(tau_Err)  "tau_Err"
  tau_des [Nm]/1 -> "Torque Limiter (outside) "/1
  Spring Stiffness/1 -> Sum2/2  "tau_L"
  Gain2/1 -> Sum3/1
  "Torque Limiter (outside) "/1 -> Gain2/1, Sum2/1
  Position PD/1(out) -> tau_cmd [Nm]/1
  Sum4/1 -> Position PD/1(position_Err)
  phi_gear [rad]/1 -> Sum4/2, Sum1/1

== system initial_setup/Simple Sinusoidal Motion/SEA Controllers (Right Leg)/SEA Controller (Position) front ==
  phi_load [rad] : Inport
  phi_gear [rad] : Inport  Port=2
  tau_des [Nm] : Inport  Port=3
  Gain2 : Gain  Gain=1/k_leg_spring
  Position PD : Subsystem
  Spring Stiffness : Gain  Gain=k_leg_spring
  Sum1 : Sum  Inputs=+-
  Sum2 : Sum  Inputs=|+-
  Sum3 : Sum  Inputs=+|+
  Sum4 : Sum  Inputs=|+-
  Sum5 : Sum  Inputs=++|
  "Torque Limiter (outside) " : Saturate  UpperLimit=LEG_MTR_MAX_TORQUE  LowerLimit=-LEG_MTR_MAX_TORQUE
  Torque PD : Subsystem
  tau_cmd [Nm] : Outport
  wires:
  phi_gear [rad]/1 -> Sum1/1, Sum4/2
  Sum4/1 -> Position PD/1(position_Err)
  Position PD/1(out) -> tau_cmd [Nm]/1
  "Torque Limiter (outside) "/1 -> Sum2/1, Gain2/1
  Gain2/1 -> Sum3/1
  Spring Stiffness/1 -> Sum2/2  "tau_L"
  tau_des [Nm]/1 -> "Torque Limiter (outside) "/1
  Sum2/1 -> Torque PD/1(tau_Err)  "tau_Err"
  Sum1/1 -> Spring Stiffness/1
  phi_load [rad]/1 -> Sum3/2, Sum1/2
  Sum3/1 -> Sum5/1
  Sum5/1 -> Sum4/1
  Torque PD/1(out) -> Sum5/2

== system initial_setup/Simple Sinusoidal Motion/SEA Controllers (Right Leg)/SEA Controller (Velocity) back ==
  note: Anticipatory Feedforward Compensation
  note: Inverse Dynamics Compensation
  note: SEA
      | Electromechanical
      | Process
      | Dynamics
  note: Feedback Error Compensation
  phi_load [rad] : Inport
  phi_gear [rad] : Inport  Port=2
  tau_des [Nm] : Inport  Port=3
  1st Lead Compensator : Subsystem
  Gain2 : Gain  Gain=1/k_leg_spring
  Gear Ratio2 : Gain  Gain=LEG_MTR_GEAR_RATIO
  Lead Compensator : Subsystem
  PD : Subsystem
  PID : Subsystem
  Spring Stiffness : Gain  Gain=k_leg_spring
  Sum1 : Sum  Inputs=+-
  Sum2 : Sum  Inputs=|+-
  Sum3 : Sum  Inputs=+|+
  Sum4 : Sum  Inputs=|+-
  Sum5 : Sum  Inputs=++|
  "Torque Limiter (outside) " : Saturate  UpperLimit=LEG_MTR_MAX_TORQUE  LowerLimit=-LEG_MTR_MAX_TORQUE
  Velocity Limiter : Saturate  UpperLimit=LEG_MTR_MAX_VELOCITY  LowerLimit=-LEG_MTR_MAX_VELOCITY
  filtered_derivative : Subsystem
  tau_cmd [Nm] : Outport
  wires:
  Gain2/1 -> 1st Lead Compensator/1(x)
  phi_load [rad]/1 -> Lead Compensator/1(x), Sum1/2
  Sum1/1 -> Spring Stiffness/1
  Sum2/1 -> PID/1(tau_Err)  "tau_Err"
  tau_des [Nm]/1 -> "Torque Limiter (outside) "/1
  Spring Stiffness/1 -> Sum2/2  "tau_L"
  PID/1("dphi_gearhead_des [rad/s] ") -> Sum5/2
  1st Lead Compensator/1(dx/dt) -> Sum3/1
  phi_gear [rad]/1 -> filtered_derivative/1(x), Sum1/1
  Sum5/1 -> Velocity Limiter/1  "dphi_gearhead_des  [m/s]"
  "Torque Limiter (outside) "/1 -> Sum2/1, Gain2/1
  Lead Compensator/1(dx/dt) -> Sum3/2
  Velocity Limiter/1 -> Sum4/1
  Sum4/1 -> PD/1(velocity_err [rad/s])
  filtered_derivative/1(dx/dt) -> Gear Ratio2/1
  Gear Ratio2/1 -> Sum4/2
  Sum3/1 -> Sum5/1
  PD/1(tau_mtr [Nm]) -> tau_cmd [Nm]/1

== system initial_setup/Simple Sinusoidal Motion/SEA Controllers (Right Leg)/SEA Controller (Velocity) front ==
  note: Feedback Error Compensation
  note: SEA
      | Electromechanical
      | Process
      | Dynamics
  note: Inverse Dynamics Compensation
  note: Anticipatory Feedforward Compensation
  phi_load [rad] : Inport
  phi_gear [rad] : Inport  Port=2
  tau_des [Nm] : Inport  Port=3
  1st Lead Compensator : Subsystem
  Gain2 : Gain  Gain=1/k_leg_spring
  Gear Ratio2 : Gain  Gain=LEG_MTR_GEAR_RATIO
  Lead Compensator : Subsystem
  PD : Subsystem
  PID : Subsystem
  Spring Stiffness : Gain  Gain=k_leg_spring
  Sum1 : Sum  Inputs=+-
  Sum2 : Sum  Inputs=|+-
  Sum3 : Sum  Inputs=+|+
  Sum4 : Sum  Inputs=|+-
  Sum5 : Sum  Inputs=++|
  "Torque Limiter (outside) " : Saturate  UpperLimit=LEG_MTR_MAX_TORQUE  LowerLimit=-LEG_MTR_MAX_TORQUE
  Velocity Limiter : Saturate  UpperLimit=LEG_MTR_MAX_VELOCITY  LowerLimit=-LEG_MTR_MAX_VELOCITY
  filtered_derivative : Subsystem
  tau_cmd [Nm] : Outport
  wires:
  PD/1(tau_mtr [Nm]) -> tau_cmd [Nm]/1
  Sum3/1 -> Sum5/1
  Gear Ratio2/1 -> Sum4/2
  filtered_derivative/1(dx/dt) -> Gear Ratio2/1
  Sum4/1 -> PD/1(velocity_err [rad/s])
  Velocity Limiter/1 -> Sum4/1
  Lead Compensator/1(dx/dt) -> Sum3/2
  "Torque Limiter (outside) "/1 -> Gain2/1, Sum2/1
  Sum5/1 -> Velocity Limiter/1  "dphi_gearhead_des  [m/s]"
  phi_gear [rad]/1 -> Sum1/1, filtered_derivative/1(x)
  1st Lead Compensator/1(dx/dt) -> Sum3/1
  PID/1("dphi_gearhead_des [rad/s] ") -> Sum5/2
  Spring Stiffness/1 -> Sum2/2  "tau_L"
  tau_des [Nm]/1 -> "Torque Limiter (outside) "/1
  Sum2/1 -> PID/1(tau_Err)  "tau_Err"
  Sum1/1 -> Spring Stiffness/1
  phi_load [rad]/1 -> Sum1/2, Lead Compensator/1(x)
  Gain2/1 -> 1st Lead Compensator/1(x)

== system initial_setup/Simple Sinusoidal Motion/SEA Controllers (Left Leg)/SEA Controller (Position) back/Position PD ==
  position_Err : Inport
  Proportional Gain : Gain  Gain=kp_sea_position
  Proportional Gain1 : Gain  Gain=kd_sea_position
  Sum : Sum
  filtered_derivative : Subsystem
  out : Outport
  wires:
  filtered_derivative/1(dx/dt) -> Proportional Gain1/1
  Proportional Gain1/1 -> Sum/1
  Proportional Gain/1 -> Sum/2
  position_Err/1 -> Proportional Gain/1, filtered_derivative/1(x)
  Sum/1 -> out/1

== system initial_setup/Simple Sinusoidal Motion/SEA Controllers (Left Leg)/SEA Controller (Position) back/Torque PD ==
  tau_Err : Inport
  Proportional Gain : Gain  Gain=kp_sea_torque
  out : Outport
  wires:
  Proportional Gain/1 -> out/1
  tau_Err/1 -> Proportional Gain/1

== system initial_setup/Simple Sinusoidal Motion/SEA Controllers (Left Leg)/SEA Controller (Position) front/Position PD ==
  position_Err : Inport
  Proportional Gain : Gain  Gain=kp_sea_position
  Proportional Gain1 : Gain  Gain=kd_sea_position
  Sum : Sum
  filtered_derivative : Subsystem
  out : Outport
  wires:
  filtered_derivative/1(dx/dt) -> Proportional Gain1/1
  Sum/1 -> out/1
  position_Err/1 -> Proportional Gain/1, filtered_derivative/1(x)
  Proportional Gain/1 -> Sum/2
  Proportional Gain1/1 -> Sum/1

== system initial_setup/Simple Sinusoidal Motion/SEA Controllers (Left Leg)/SEA Controller (Position) front/Torque PD ==
  tau_Err : Inport
  Proportional Gain : Gain  Gain=kp_sea_torque
  out : Outport
  wires:
  tau_Err/1 -> Proportional Gain/1
  Proportional Gain/1 -> out/1

== system initial_setup/Simple Sinusoidal Motion/SEA Controllers (Left Leg)/SEA Controller (Velocity) back/1st Lead Compensator ==
  x : Inport
  Gain1 : Gain  Gain=1/sample_time
  difference : simulink/Discrete/Difference  ICPrevInput=0.0  InputProcessing=Inherited  OutMin=[]  OutMax=[]  OutDataType=fixdt(1, 16)  OutScaling=2^-10  DoSatur=off
  single_pole_filter : DiscreteTransferFcn  Numerator=[(1-exp(-2*pi*fcut_velocity*sample_time)) 0]  Denominator=[1 -exp(-2*pi*fcut_velocity*sample_time)]  SampleTime=sample_time
  dx/dt : Outport
  wires:
  x/1 -> difference/1
  single_pole_filter/1 -> dx/dt/1
  difference/1 -> Gain1/1
  Gain1/1 -> single_pole_filter/1

== system initial_setup/Simple Sinusoidal Motion/SEA Controllers (Left Leg)/SEA Controller (Velocity) back/Lead Compensator ==
  x : Inport
  Gain1 : Gain  Gain=1/sample_time
  difference : simulink/Discrete/Difference  ICPrevInput=0.0  InputProcessing=Inherited  OutMin=[]  OutMax=[]  OutDataType=fixdt(1, 16)  OutScaling=2^-10  DoSatur=off
  single_pole_filter : DiscreteTransferFcn  Numerator=[(1-exp(-2*pi*fcut_velocity*sample_time)) 0]  Denominator=[1 -exp(-2*pi*fcut_velocity*sample_time)]  SampleTime=sample_time
  dx/dt : Outport
  wires:
  x/1 -> difference/1
  single_pole_filter/1 -> dx/dt/1
  difference/1 -> Gain1/1
  Gain1/1 -> single_pole_filter/1

== system initial_setup/Simple Sinusoidal Motion/SEA Controllers (Left Leg)/SEA Controller (Velocity) back/PD ==
  velocity_err [rad/s] : Inport
  Derivative Gain : Gain  Gain=kd_velocity
  Proportional Gain : Gain  Gain=kp_velocity
  Sum : Sum
  filtered_derivative : Subsystem
  tau_mtr [Nm] : Outport
  wires:
  velocity_err [rad/s]/1 -> Proportional Gain/1, filtered_derivative/1(x)
  Proportional Gain/1 -> Sum/1
  Derivative Gain/1 -> Sum/2
  Sum/1 -> tau_mtr [Nm]/1
  filtered_derivative/1(dx/dt) -> Derivative Gain/1

== system initial_setup/Simple Sinusoidal Motion/SEA Controllers (Left Leg)/SEA Controller (Velocity) back/PID ==
  tau_Err : Inport
  Proportional Gain : Gain  Gain=kp_sea_torque
  Proportional Gain1 : Gain  Gain=kd_sea_torque
  Sum : Sum
  filtered_derivative : Subsystem
  "dphi_gearhead_des [rad/s] " : Outport
  wires:
  Sum/1 -> "dphi_gearhead_des [rad/s] "/1
  tau_Err/1 -> Proportional Gain/1, filtered_derivative/1(x)
  Proportional Gain/1 -> Sum/2
  Proportional Gain1/1 -> Sum/1
  filtered_derivative/1(dx/dt) -> Proportional Gain1/1

== system initial_setup/Simple Sinusoidal Motion/SEA Controllers (Left Leg)/SEA Controller (Velocity) back/filtered_derivative ==
  x : Inport
  Gain1 : Gain  Gain=1/sample_time
  difference : simulink/Discrete/Difference  ICPrevInput=0.0  InputProcessing=Inherited  OutMin=[]  OutMax=[]  OutDataType=fixdt(1, 16)  OutScaling=2^-10  DoSatur=off
  single_pole_filter : DiscreteTransferFcn  Numerator=[(1-exp(-2*pi*fcut_velocity*sample_time)) 0]  Denominator=[1 -exp(-2*pi*fcut_velocity*sample_time)]  SampleTime=sample_time
  dx/dt : Outport
  wires:
  x/1 -> difference/1
  single_pole_filter/1 -> dx/dt/1
  difference/1 -> Gain1/1
  Gain1/1 -> single_pole_filter/1

== system initial_setup/Simple Sinusoidal Motion/SEA Controllers (Left Leg)/SEA Controller (Velocity) front/1st Lead Compensator ==
  x : Inport
  Gain1 : Gain  Gain=1/sample_time
  difference : simulink/Discrete/Difference  ICPrevInput=0.0  InputProcessing=Inherited  OutMin=[]  OutMax=[]  OutDataType=fixdt(1, 16)  OutScaling=2^-10  DoSatur=off
  single_pole_filter : DiscreteTransferFcn  Numerator=[(1-exp(-2*pi*fcut_velocity*sample_time)) 0]  Denominator=[1 -exp(-2*pi*fcut_velocity*sample_time)]  SampleTime=sample_time
  dx/dt : Outport
  wires:
  Gain1/1 -> single_pole_filter/1
  difference/1 -> Gain1/1
  single_pole_filter/1 -> dx/dt/1
  x/1 -> difference/1

== system initial_setup/Simple Sinusoidal Motion/SEA Controllers (Left Leg)/SEA Controller (Velocity) front/Lead Compensator ==
  x : Inport
  Gain1 : Gain  Gain=1/sample_time
  difference : simulink/Discrete/Difference  ICPrevInput=0.0  InputProcessing=Inherited  OutMin=[]  OutMax=[]  OutDataType=fixdt(1, 16)  OutScaling=2^-10  DoSatur=off
  single_pole_filter : DiscreteTransferFcn  Numerator=[(1-exp(-2*pi*fcut_velocity*sample_time)) 0]  Denominator=[1 -exp(-2*pi*fcut_velocity*sample_time)]  SampleTime=sample_time
  dx/dt : Outport
  wires:
  Gain1/1 -> single_pole_filter/1
  difference/1 -> Gain1/1
  single_pole_filter/1 -> dx/dt/1
  x/1 -> difference/1

== system initial_setup/Simple Sinusoidal Motion/SEA Controllers (Left Leg)/SEA Controller (Velocity) front/PD ==
  velocity_err [rad/s] : Inport
  Derivative Gain : Gain  Gain=kd_velocity
  Proportional Gain : Gain  Gain=kp_velocity
  Sum : Sum
  filtered_derivative : Subsystem
  tau_mtr [Nm] : Outport
  wires:
  filtered_derivative/1(dx/dt) -> Derivative Gain/1
  Sum/1 -> tau_mtr [Nm]/1
  Derivative Gain/1 -> Sum/2
  Proportional Gain/1 -> Sum/1
  velocity_err [rad/s]/1 -> filtered_derivative/1(x), Proportional Gain/1

== system initial_setup/Simple Sinusoidal Motion/SEA Controllers (Left Leg)/SEA Controller (Velocity) front/PID ==
  tau_Err : Inport
  Proportional Gain : Gain  Gain=kp_sea_torque
  Proportional Gain1 : Gain  Gain=kd_sea_torque
  Sum : Sum
  filtered_derivative : Subsystem
  "dphi_gearhead_des [rad/s] " : Outport
  wires:
  filtered_derivative/1(dx/dt) -> Proportional Gain1/1
  Proportional Gain1/1 -> Sum/1
  Proportional Gain/1 -> Sum/2
  tau_Err/1 -> filtered_derivative/1(x), Proportional Gain/1
  Sum/1 -> "dphi_gearhead_des [rad/s] "/1

== system initial_setup/Simple Sinusoidal Motion/SEA Controllers (Left Leg)/SEA Controller (Velocity) front/filtered_derivative ==
  x : Inport
  Gain1 : Gain  Gain=1/sample_time
  difference : simulink/Discrete/Difference  ICPrevInput=0.0  InputProcessing=Inherited  OutMin=[]  OutMax=[]  OutDataType=fixdt(1, 16)  OutScaling=2^-10  DoSatur=off
  single_pole_filter : DiscreteTransferFcn  Numerator=[(1-exp(-2*pi*fcut_velocity*sample_time)) 0]  Denominator=[1 -exp(-2*pi*fcut_velocity*sample_time)]  SampleTime=sample_time
  dx/dt : Outport
  wires:
  Gain1/1 -> single_pole_filter/1
  difference/1 -> Gain1/1
  single_pole_filter/1 -> dx/dt/1
  x/1 -> difference/1

== system initial_setup/Simple Sinusoidal Motion/SEA Controllers (Right Leg)/SEA Controller (Position) back/Position PD ==
  position_Err : Inport
  Proportional Gain : Gain  Gain=kp_sea_position
  Proportional Gain1 : Gain  Gain=kd_sea_position
  Sum : Sum
  filtered_derivative : Subsystem
  out : Outport
  wires:
  Sum/1 -> out/1
  position_Err/1 -> filtered_derivative/1(x), Proportional Gain/1
  Proportional Gain/1 -> Sum/2
  Proportional Gain1/1 -> Sum/1
  filtered_derivative/1(dx/dt) -> Proportional Gain1/1

== system initial_setup/Simple Sinusoidal Motion/SEA Controllers (Right Leg)/SEA Controller (Position) back/Torque PD ==
  tau_Err : Inport
  Proportional Gain : Gain  Gain=kp_sea_torque
  out : Outport
  wires:
  tau_Err/1 -> Proportional Gain/1
  Proportional Gain/1 -> out/1

== system initial_setup/Simple Sinusoidal Motion/SEA Controllers (Right Leg)/SEA Controller (Position) front/Position PD ==
  position_Err : Inport
  Proportional Gain : Gain  Gain=kp_sea_position
  Proportional Gain1 : Gain  Gain=kd_sea_position
  Sum : Sum
  filtered_derivative : Subsystem
  out : Outport
  wires:
  Proportional Gain1/1 -> Sum/1
  Proportional Gain/1 -> Sum/2
  position_Err/1 -> filtered_derivative/1(x), Proportional Gain/1
  Sum/1 -> out/1
  filtered_derivative/1(dx/dt) -> Proportional Gain1/1

== system initial_setup/Simple Sinusoidal Motion/SEA Controllers (Right Leg)/SEA Controller (Position) front/Torque PD ==
  tau_Err : Inport
  Proportional Gain : Gain  Gain=kp_sea_torque
  out : Outport
  wires:
  Proportional Gain/1 -> out/1
  tau_Err/1 -> Proportional Gain/1

== system initial_setup/Simple Sinusoidal Motion/SEA Controllers (Right Leg)/SEA Controller (Velocity) back/1st Lead Compensator ==
  x : Inport
  Gain1 : Gain  Gain=1/sample_time
  difference : simulink/Discrete/Difference  ICPrevInput=0.0  InputProcessing=Inherited  OutMin=[]  OutMax=[]  OutDataType=fixdt(1, 16)  OutScaling=2^-10  DoSatur=off
  single_pole_filter : DiscreteTransferFcn  Numerator=[(1-exp(-2*pi*fcut_velocity*sample_time)) 0]  Denominator=[1 -exp(-2*pi*fcut_velocity*sample_time)]  SampleTime=sample_time
  dx/dt : Outport
  wires:
  Gain1/1 -> single_pole_filter/1
  difference/1 -> Gain1/1
  single_pole_filter/1 -> dx/dt/1
  x/1 -> difference/1

== system initial_setup/Simple Sinusoidal Motion/SEA Controllers (Right Leg)/SEA Controller (Velocity) back/Lead Compensator ==
  x : Inport
  Gain1 : Gain  Gain=1/sample_time
  difference : simulink/Discrete/Difference  ICPrevInput=0.0  InputProcessing=Inherited  OutMin=[]  OutMax=[]  OutDataType=fixdt(1, 16)  OutScaling=2^-10  DoSatur=off
  single_pole_filter : DiscreteTransferFcn  Numerator=[(1-exp(-2*pi*fcut_velocity*sample_time)) 0]  Denominator=[1 -exp(-2*pi*fcut_velocity*sample_time)]  SampleTime=sample_time
  dx/dt : Outport
  wires:
  Gain1/1 -> single_pole_filter/1
  difference/1 -> Gain1/1
  single_pole_filter/1 -> dx/dt/1
  x/1 -> difference/1

== system initial_setup/Simple Sinusoidal Motion/SEA Controllers (Right Leg)/SEA Controller (Velocity) back/PD ==
  velocity_err [rad/s] : Inport
  Derivative Gain : Gain  Gain=kd_velocity
  Proportional Gain : Gain  Gain=kp_velocity
  Sum : Sum
  filtered_derivative : Subsystem
  tau_mtr [Nm] : Outport
  wires:
  filtered_derivative/1(dx/dt) -> Derivative Gain/1
  Sum/1 -> tau_mtr [Nm]/1
  Derivative Gain/1 -> Sum/2
  Proportional Gain/1 -> Sum/1
  velocity_err [rad/s]/1 -> filtered_derivative/1(x), Proportional Gain/1

== system initial_setup/Simple Sinusoidal Motion/SEA Controllers (Right Leg)/SEA Controller (Velocity) back/PID ==
  tau_Err : Inport
  Proportional Gain : Gain  Gain=kp_sea_torque
  Proportional Gain1 : Gain  Gain=kd_sea_torque
  Sum : Sum
  filtered_derivative : Subsystem
  "dphi_gearhead_des [rad/s] " : Outport
  wires:
  filtered_derivative/1(dx/dt) -> Proportional Gain1/1
  Proportional Gain1/1 -> Sum/1
  Proportional Gain/1 -> Sum/2
  tau_Err/1 -> filtered_derivative/1(x), Proportional Gain/1
  Sum/1 -> "dphi_gearhead_des [rad/s] "/1

== system initial_setup/Simple Sinusoidal Motion/SEA Controllers (Right Leg)/SEA Controller (Velocity) back/filtered_derivative ==
  x : Inport
  Gain1 : Gain  Gain=1/sample_time
  difference : simulink/Discrete/Difference  ICPrevInput=0.0  InputProcessing=Inherited  OutMin=[]  OutMax=[]  OutDataType=fixdt(1, 16)  OutScaling=2^-10  DoSatur=off
  single_pole_filter : DiscreteTransferFcn  Numerator=[(1-exp(-2*pi*fcut_velocity*sample_time)) 0]  Denominator=[1 -exp(-2*pi*fcut_velocity*sample_time)]  SampleTime=sample_time
  dx/dt : Outport
  wires:
  Gain1/1 -> single_pole_filter/1
  difference/1 -> Gain1/1
  single_pole_filter/1 -> dx/dt/1
  x/1 -> difference/1

== system initial_setup/Simple Sinusoidal Motion/SEA Controllers (Right Leg)/SEA Controller (Velocity) front/1st Lead Compensator ==
  x : Inport
  Gain1 : Gain  Gain=1/sample_time
  difference : simulink/Discrete/Difference  ICPrevInput=0.0  InputProcessing=Inherited  OutMin=[]  OutMax=[]  OutDataType=fixdt(1, 16)  OutScaling=2^-10  DoSatur=off
  single_pole_filter : DiscreteTransferFcn  Numerator=[(1-exp(-2*pi*fcut_velocity*sample_time)) 0]  Denominator=[1 -exp(-2*pi*fcut_velocity*sample_time)]  SampleTime=sample_time
  dx/dt : Outport
  wires:
  x/1 -> difference/1
  single_pole_filter/1 -> dx/dt/1
  difference/1 -> Gain1/1
  Gain1/1 -> single_pole_filter/1

== system initial_setup/Simple Sinusoidal Motion/SEA Controllers (Right Leg)/SEA Controller (Velocity) front/Lead Compensator ==
  x : Inport
  Gain1 : Gain  Gain=1/sample_time
  difference : simulink/Discrete/Difference  ICPrevInput=0.0  InputProcessing=Inherited  OutMin=[]  OutMax=[]  OutDataType=fixdt(1, 16)  OutScaling=2^-10  DoSatur=off
  single_pole_filter : DiscreteTransferFcn  Numerator=[(1-exp(-2*pi*fcut_velocity*sample_time)) 0]  Denominator=[1 -exp(-2*pi*fcut_velocity*sample_time)]  SampleTime=sample_time
  dx/dt : Outport
  wires:
  x/1 -> difference/1
  single_pole_filter/1 -> dx/dt/1
  difference/1 -> Gain1/1
  Gain1/1 -> single_pole_filter/1

== system initial_setup/Simple Sinusoidal Motion/SEA Controllers (Right Leg)/SEA Controller (Velocity) front/PD ==
  velocity_err [rad/s] : Inport
  Derivative Gain : Gain  Gain=kd_velocity
  Proportional Gain : Gain  Gain=kp_velocity
  Sum : Sum
  filtered_derivative : Subsystem
  tau_mtr [Nm] : Outport
  wires:
  velocity_err [rad/s]/1 -> Proportional Gain/1, filtered_derivative/1(x)
  Proportional Gain/1 -> Sum/1
  Derivative Gain/1 -> Sum/2
  Sum/1 -> tau_mtr [Nm]/1
  filtered_derivative/1(dx/dt) -> Derivative Gain/1

== system initial_setup/Simple Sinusoidal Motion/SEA Controllers (Right Leg)/SEA Controller (Velocity) front/PID ==
  tau_Err : Inport
  Proportional Gain : Gain  Gain=kp_sea_torque
  Proportional Gain1 : Gain  Gain=kd_sea_torque
  Sum : Sum
  filtered_derivative : Subsystem
  "dphi_gearhead_des [rad/s] " : Outport
  wires:
  Sum/1 -> "dphi_gearhead_des [rad/s] "/1
  tau_Err/1 -> Proportional Gain/1, filtered_derivative/1(x)
  Proportional Gain/1 -> Sum/2
  Proportional Gain1/1 -> Sum/1
  filtered_derivative/1(dx/dt) -> Proportional Gain1/1

== system initial_setup/Simple Sinusoidal Motion/SEA Controllers (Right Leg)/SEA Controller (Velocity) front/filtered_derivative ==
  x : Inport
  Gain1 : Gain  Gain=1/sample_time
  difference : simulink/Discrete/Difference  ICPrevInput=0.0  InputProcessing=Inherited  OutMin=[]  OutMax=[]  OutDataType=fixdt(1, 16)  OutScaling=2^-10  DoSatur=off
  single_pole_filter : DiscreteTransferFcn  Numerator=[(1-exp(-2*pi*fcut_velocity*sample_time)) 0]  Denominator=[1 -exp(-2*pi*fcut_velocity*sample_time)]  SampleTime=sample_time
  dx/dt : Outport
  wires:
  x/1 -> difference/1
  single_pole_filter/1 -> dx/dt/1
  difference/1 -> Gain1/1
  Gain1/1 -> single_pole_filter/1

== system initial_setup/Simple Sinusoidal Motion/SEA Controllers (Left Leg)/SEA Controller (Position) back/Position PD/filtered_derivative ==
  x : Inport
  Gain1 : Gain  Gain=1/sample_time
  difference : simulink/Discrete/Difference  ICPrevInput=0.0  InputProcessing=Inherited  OutMin=[]  OutMax=[]  OutDataType=fixdt(1, 16)  OutScaling=2^-10  DoSatur=off
  single_pole_filter : DiscreteTransferFcn  Numerator=[(1-exp(-2*pi*fcut_velocity*sample_time)) 0]  Denominator=[1 -exp(-2*pi*fcut_velocity*sample_time)]  SampleTime=sample_time
  dx/dt : Outport
  wires:
  x/1 -> difference/1
  single_pole_filter/1 -> dx/dt/1
  difference/1 -> Gain1/1
  Gain1/1 -> single_pole_filter/1

== system initial_setup/Simple Sinusoidal Motion/SEA Controllers (Left Leg)/SEA Controller (Position) front/Position PD/filtered_derivative ==
  x : Inport
  Gain1 : Gain  Gain=1/sample_time
  difference : simulink/Discrete/Difference  ICPrevInput=0.0  InputProcessing=Inherited  OutMin=[]  OutMax=[]  OutDataType=fixdt(1, 16)  OutScaling=2^-10  DoSatur=off
  single_pole_filter : DiscreteTransferFcn  Numerator=[(1-exp(-2*pi*fcut_velocity*sample_time)) 0]  Denominator=[1 -exp(-2*pi*fcut_velocity*sample_time)]  SampleTime=sample_time
  dx/dt : Outport
  wires:
  x/1 -> difference/1
  single_pole_filter/1 -> dx/dt/1
  difference/1 -> Gain1/1
  Gain1/1 -> single_pole_filter/1

== system initial_setup/Simple Sinusoidal Motion/SEA Controllers (Left Leg)/SEA Controller (Velocity) back/PD/filtered_derivative ==
  x : Inport
  Gain1 : Gain  Gain=1/sample_time
  difference : simulink/Discrete/Difference  ICPrevInput=0.0  InputProcessing=Inherited  OutMin=[]  OutMax=[]  OutDataType=fixdt(1, 16)  OutScaling=2^-10  DoSatur=off
  single_pole_filter : DiscreteTransferFcn  Numerator=[(1-exp(-2*pi*fcut_velocity*sample_time)) 0]  Denominator=[1 -exp(-2*pi*fcut_velocity*sample_time)]  SampleTime=sample_time
  dx/dt : Outport
  wires:
  x/1 -> difference/1
  single_pole_filter/1 -> dx/dt/1
  difference/1 -> Gain1/1
  Gain1/1 -> single_pole_filter/1

== system initial_setup/Simple Sinusoidal Motion/SEA Controllers (Left Leg)/SEA Controller (Velocity) back/PID/filtered_derivative ==
  x : Inport
  Gain1 : Gain  Gain=1/sample_time
  difference : simulink/Discrete/Difference  ICPrevInput=0.0  InputProcessing=Inherited  OutMin=[]  OutMax=[]  OutDataType=fixdt(1, 16)  OutScaling=2^-10  DoSatur=off
  single_pole_filter : DiscreteTransferFcn  Numerator=[(1-exp(-2*pi*fcut_velocity*sample_time)) 0]  Denominator=[1 -exp(-2*pi*fcut_velocity*sample_time)]  SampleTime=sample_time
  dx/dt : Outport
  wires:
  x/1 -> difference/1
  single_pole_filter/1 -> dx/dt/1
  difference/1 -> Gain1/1
  Gain1/1 -> single_pole_filter/1

== system initial_setup/Simple Sinusoidal Motion/SEA Controllers (Left Leg)/SEA Controller (Velocity) front/PD/filtered_derivative ==
  x : Inport
  Gain1 : Gain  Gain=1/sample_time
  difference : simulink/Discrete/Difference  ICPrevInput=0.0  InputProcessing=Inherited  OutMin=[]  OutMax=[]  OutDataType=fixdt(1, 16)  OutScaling=2^-10  DoSatur=off
  single_pole_filter : DiscreteTransferFcn  Numerator=[(1-exp(-2*pi*fcut_velocity*sample_time)) 0]  Denominator=[1 -exp(-2*pi*fcut_velocity*sample_time)]  SampleTime=sample_time
  dx/dt : Outport
  wires:
  Gain1/1 -> single_pole_filter/1
  difference/1 -> Gain1/1
  single_pole_filter/1 -> dx/dt/1
  x/1 -> difference/1
